simulink model "Eas_Integrated_Harness"  (R2021a)
settings: Solver=FixedStepDiscrete  StartTime=0.0  StopTime=inf  FixedStep=0.01  RelTol=1e-3
settings Model: DataDictionary=DPF_Data_Dictionary.sldd  Creator=SOMNATH  LastModifiedBy=SOMNATH
settings OptimizationCC: BlockReduction=off  DefaultParameterBehavior=Inlined  UseDivisionForNetSlopeComputation=on  EnhancedBackFolding=on  PassReuseOutputArgsAs=Individual arguments  EfficientFloat2IntCast=on  LifeSpan=Inf  OptimizeBlockOrder=speed  DifferentSizesBufferReuse=on  OptimizationCustomize=off  EfficientTunableParamExpr=on
settings DebuggingCC: SignalInfNanChecking=error  SignalRangeChecking=error  ReadBeforeWriteMsg=EnableAllAsError  WriteAfterWriteMsg=EnableAllAsError  WriteAfterReadMsg=EnableAllAsError  AlgebraicLoopMsg=error  ArtificialAlgebraicLoopMsg=error  SaveWithDisabledLinksMsg=error  SaveWithParameterizedLinksMsg=error  BlockPriorityViolationMsg=error  SolverPrmCheckMsg=error  InheritedTsInSrcMsg=error  SingleTaskRateTransMsg=error  TasksWithSamePriorityMsg=error  SigSpecEnsureSampleTimeMsg=error  CheckMatrixSingularityMsg=error  IntegerOverflowMsg=error  ParameterUnderflowMsg=error  ParameterPrecisionLossMsg=error  ParameterTunabilityLossMsg=error  UnderSpecifiedDataTypeMsg=error  UnnecessaryDatatypeConvMsg=warning  VectorMatrixConversionMsg=error  SignalLabelMismatchMsg=error  UnconnectedInputMsg=error  UnconnectedOutputMsg=error  UnconnectedLineMsg=error  SFcnCompatibilityMsg=error  UniqueDataStoreMsg=error  BusObjectLabelMismatch=error  RootOutportRequireBusObject=error  AssertControl=DisableAll  ModelReferenceIOMsg=error  ModelReferenceIOMismatchMessage=error  UnknownTsInhSupMsg=error  ModelReferenceDataLoggingMessage=error  StateNameClashWarn=warning  StrictBusMsg=ErrorOnBusTreatedAsVector  NonBusSignalsTreatedAsBus=error  SFInvalidInputDataAccessInChartInitDiag=error  SFTransitionOutsideNaturalParentDiag=error  SFUnreachableExecutionPathDiag=error  SFUndirectedBroadcastEventsDiag=error  SFTransitionActionBeforeConditionDiag=error  SFTemporalDelaySmallerThanSampleTimeDiag=error  SFSelfTransitionDiag=error  SFExecutionAtInitializationDiag=error  IntegerSaturationMsg=error
settings SFSimCC: CompileTimeRecursionLimit=0  EnableRuntimeRecursion=off  MATLABDynamicMemAlloc=off
settings RTWCC: SystemTargetFile=ert.tlc  GenCodeOnly=on  TemplateMakefile=ert_default_tmf  GenerateReport=on  Toolchain=MinGW64 | gmake (64-bit Windows)  IncludeHyperlinkInReport=on  LaunchReport=on  GenerateTraceInfo=on  GenerateTraceReport=on  GenerateTraceReportSl=on  GenerateTraceReportSf=on  GenerateTraceReportEml=on  GenerateWebview=on  GenerateCodeReplacementReport=on
settings CodeAppCC: ForceParamTrailComments=on  IgnoreCustomStorageClasses=off  OperatorAnnotations=on  SimulinkDataObjDesc=on  SFDataObjDesc=on  MATLABFcnDesc=on  MangleLength=4  InsertBlockDesc=on  ReqsInCode=on
settings ERTTargetCC: TargetLangStandard=C99 (ISO)  UtilityFuncGeneration=Shared location  GenerateSampleERTMain=on  IncludeMdlTerminateFcn=off  SuppressErrorStatus=on  SupportAbsoluteTime=off  SupportNonFinite=off  ParenthesesLevel=Maximum  CastingMode=Standards  GenerateSharedConstants=off  InlinedParameterPlacement=NonHierarchical  ERTCustomFileTemplate=example_file_process.tlc  PreserveExpressionOrder=on  EnableSignedLeftShifts=off  EnableSignedRightShifts=off
settings ConfigComp: CovMetricSettings=dcmwe  DVMode=PropertyProving  DVTestSuiteOptimization=Auto  DVDetectDeadLogic=on  DVDetectActiveLogic=on  DVDetectOutOfBounds=on  DVDetectInfNaN=on  DVDesignMinMaxCheck=on  DVDetectDSMAccessViolations=on  DVDetectHISMViolationsHisl_0002=on  DVDetectHISMViolationsHisl_0003=on  DVDetectHISMViolationsHisl_0004=on  DVDetectHISMViolationsHisl_0028=on  DVDetectBlockInputRangeViolations=on  DVSaveExpectedOutput=on  DVRandomizeNoEffectData=on  DVSaveHarnessModel=on

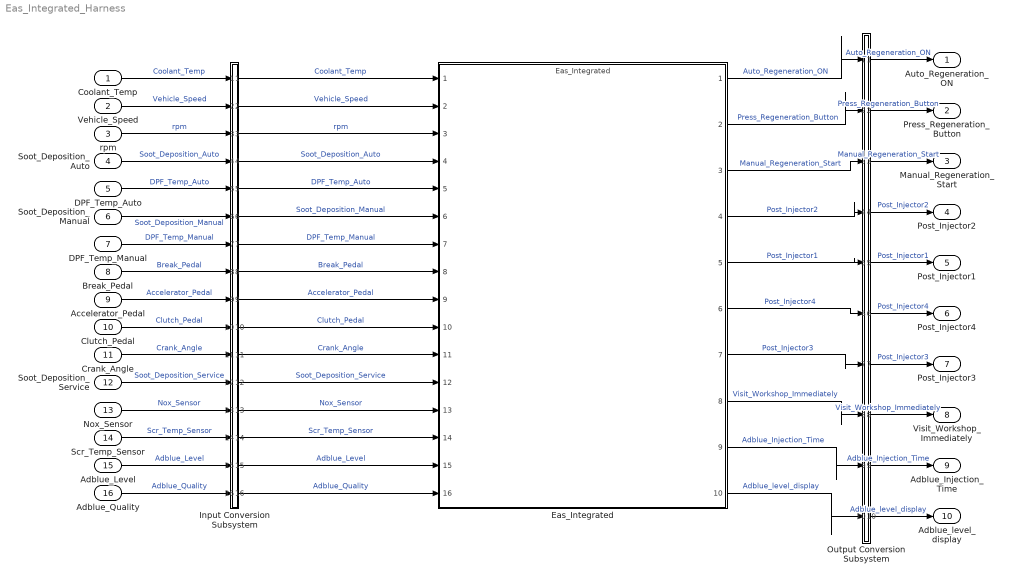
== system Eas_Integrated_Harness ==
  Coolant_Temp : Inport  OutDataTypeStr=int16  PortDimensions=[1]  SampleTime=0.01
  Vehicle_Speed : Inport  Port=2  OutDataTypeStr=uint8  PortDimensions=[1]  SampleTime=0.01
  rpm : Inport  Port=3  OutDataTypeStr=uint16  PortDimensions=[1]  SampleTime=0.01
  Soot_Deposition_Auto : Inport  Port=4  OutDataTypeStr=uint8  PortDimensions=[1]  SampleTime=0.01
  DPF_Temp_Auto : Inport  Port=5  OutDataTypeStr=uint8  PortDimensions=[1]  SampleTime=0.01
  Soot_Deposition_Manual : Inport  Port=6  OutDataTypeStr=uint8  PortDimensions=[1]  SampleTime=0.01
  DPF_Temp_Manual : Inport  Port=7  OutDataTypeStr=int16  PortDimensions=[1]  SampleTime=0.01
  Break_Pedal : Inport  Port=8  OutDataTypeStr=boolean  PortDimensions=[1]  SampleTime=0.01
  Accelerator_Pedal : Inport  Port=9  OutDataTypeStr=boolean  PortDimensions=[1]  SampleTime=0.01
  Clutch_Pedal : Inport  Port=10  OutDataTypeStr=boolean  PortDimensions=[1]  SampleTime=0.01
  Crank_Angle : Inport  Port=11  OutDataTypeStr=uint16  PortDimensions=[1]  SampleTime=0.01
  Soot_Deposition_Service : Inport  Port=12  OutDataTypeStr=uint8  PortDimensions=[1]  SampleTime=0.01
  Nox_Sensor : Inport  Port=13  OutDataTypeStr=uint16  PortDimensions=[1]  SampleTime=0.01
  Scr_Temp_Sensor : Inport  Port=14  OutDataTypeStr=uint16  PortDimensions=[1]  SampleTime=0.01
  Adblue_Level : Inport  Port=15  OutDataTypeStr=uint8  PortDimensions=[1]  SampleTime=0.01
  Adblue_Quality : Inport  Port=16  OutDataTypeStr=double  PortDimensions=[1]  SampleTime=0.01
  Eas_Integrated : ModelReference  ModelNameDialog=Eas_Integrated  SimulationMode=Normal  ModelReferenceVersion=1.57
  Input Conversion Subsystem : Subsystem  Tag=__SLT_ICS__  Description=|
      | Signal spec.
      | and routing
      settings: AttributesFormatString=%<Description>
  Output Conversion Subsystem : Subsystem  Tag=__SLT_OCS__  Description=|
      | Signal spec.
      | and routing
      settings: AttributesFormatString=%<Description>
  Auto_Regeneration_ON : Outport
  Press_Regeneration_Button : Outport  Port=2
  Manual_Regeneration_Start : Outport  Port=3
  Post_Injector2 : Outport  Port=4
  Post_Injector1 : Outport  Port=5
  Post_Injector4 : Outport  Port=6
  Post_Injector3 : Outport  Port=7
  Visit_Workshop_Immediately : Outport  Port=8
  Adblue_Injection_Time : Outport  Port=9
  Adblue_level_display : Outport  Port=10
  wires:
  Coolant_Temp/1 -> Input Conversion Subsystem/1(Inport_1)  "Coolant_Temp"
  Vehicle_Speed/1 -> Input Conversion Subsystem/2(Inport_2)  "Vehicle_Speed"
  rpm/1 -> Input Conversion Subsystem/3(Inport_3)  "rpm"
  Soot_Deposition_Auto/1 -> Input Conversion Subsystem/4(Inport_4)  "Soot_Deposition_Auto"
  DPF_Temp_Auto/1 -> Input Conversion Subsystem/5(Inport_5)  "DPF_Temp_Auto"
  Soot_Deposition_Manual/1 -> Input Conversion Subsystem/6(Inport_6)  "Soot_Deposition_Manual"
  DPF_Temp_Manual/1 -> Input Conversion Subsystem/7(Inport_7)  "DPF_Temp_Manual"
  Break_Pedal/1 -> Input Conversion Subsystem/8(Inport_8)  "Break_Pedal"
  Accelerator_Pedal/1 -> Input Conversion Subsystem/9(Inport_9)  "Accelerator_Pedal"
  Clutch_Pedal/1 -> Input Conversion Subsystem/10(Inport_10)  "Clutch_Pedal"
  Crank_Angle/1 -> Input Conversion Subsystem/11(Inport_11)  "Crank_Angle"
  Soot_Deposition_Service/1 -> Input Conversion Subsystem/12(Inport_12)  "Soot_Deposition_Service"
  Nox_Sensor/1 -> Input Conversion Subsystem/13(Inport_13)  "Nox_Sensor"
  Scr_Temp_Sensor/1 -> Input Conversion Subsystem/14(Inport_14)  "Scr_Temp_Sensor"
  Adblue_Level/1 -> Input Conversion Subsystem/15(Inport_15)  "Adblue_Level"
  Adblue_Quality/1 -> Input Conversion Subsystem/16(Inport_16)  "Adblue_Quality"
  Output Conversion Subsystem/1(Outport_1) -> Auto_Regeneration_ON/1  "Auto_Regeneration_ON"
  Output Conversion Subsystem/2(Outport_2) -> Press_Regeneration_Button/1  "Press_Regeneration_Button"
  Output Conversion Subsystem/3(Outport_3) -> Manual_Regeneration_Start/1  "Manual_Regeneration_Start"
  Output Conversion Subsystem/4(Outport_4) -> Post_Injector2/1  "Post_Injector2"
  Output Conversion Subsystem/5(Outport_5) -> Post_Injector1/1  "Post_Injector1"
  Output Conversion Subsystem/6(Outport_6) -> Post_Injector4/1  "Post_Injector4"
  Output Conversion Subsystem/7(Outport_7) -> Post_Injector3/1  "Post_Injector3"
  Output Conversion Subsystem/8(Outport_8) -> Visit_Workshop_Immediately/1  "Visit_Workshop_Immediately"
  Output Conversion Subsystem/9(Outport_9) -> Adblue_Injection_Time/1  "Adblue_Injection_Time"
  Output Conversion Subsystem/10(Outport_10) -> Adblue_level_display/1  "Adblue_level_display"
  Input Conversion Subsystem/1(Outport_1) -> Eas_Integrated/1  "Coolant_Temp"
  Input Conversion Subsystem/2(Outport_2) -> Eas_Integrated/2  "Vehicle_Speed"
  Input Conversion Subsystem/3(Outport_3) -> Eas_Integrated/3  "rpm"
  Input Conversion Subsystem/4(Outport_4) -> Eas_Integrated/4  "Soot_Deposition_Auto"
  Input Conversion Subsystem/5(Outport_5) -> Eas_Integrated/5  "DPF_Temp_Auto"
  Input Conversion Subsystem/6(Outport_6) -> Eas_Integrated/6  "Soot_Deposition_Manual"
  Input Conversion Subsystem/7(Outport_7) -> Eas_Integrated/7  "DPF_Temp_Manual"
  Input Conversion Subsystem/8(Outport_8) -> Eas_Integrated/8  "Break_Pedal"
  Input Conversion Subsystem/9(Outport_9) -> Eas_Integrated/9  "Accelerator_Pedal"
  Input Conversion Subsystem/10(Outport_10) -> Eas_Integrated/10  "Clutch_Pedal"
  Input Conversion Subsystem/11(Outport_11) -> Eas_Integrated/11  "Crank_Angle"
  Input Conversion Subsystem/12(Outport_12) -> Eas_Integrated/12  "Soot_Deposition_Service"
  Input Conversion Subsystem/13(Outport_13) -> Eas_Integrated/13  "Nox_Sensor"
  Input Conversion Subsystem/14(Outport_14) -> Eas_Integrated/14  "Scr_Temp_Sensor"
  Input Conversion Subsystem/15(Outport_15) -> Eas_Integrated/15  "Adblue_Level"
  Input Conversion Subsystem/16(Outport_16) -> Eas_Integrated/16  "Adblue_Quality"
  Eas_Integrated/1 -> Output Conversion Subsystem/1(Inport_1)  "Auto_Regeneration_ON"
  Eas_Integrated/2 -> Output Conversion Subsystem/2(Inport_2)  "Press_Regeneration_Button"
  Eas_Integrated/3 -> Output Conversion Subsystem/3(Inport_3)  "Manual_Regeneration_Start"
  Eas_Integrated/4 -> Output Conversion Subsystem/4(Inport_4)  "Post_Injector2"
  Eas_Integrated/5 -> Output Conversion Subsystem/5(Inport_5)  "Post_Injector1"
  Eas_Integrated/6 -> Output Conversion Subsystem/6(Inport_6)  "Post_Injector4"
  Eas_Integrated/7 -> Output Conversion Subsystem/7(Inport_7)  "Post_Injector3"
  Eas_Integrated/8 -> Output Conversion Subsystem/8(Inport_8)  "Visit_Workshop_Immediately"
  Eas_Integrated/9 -> Output Conversion Subsystem/9(Inport_9)  "Adblue_Injection_Time"
  Eas_Integrated/10 -> Output Conversion Subsystem/10(Inport_10)  "Adblue_level_display"

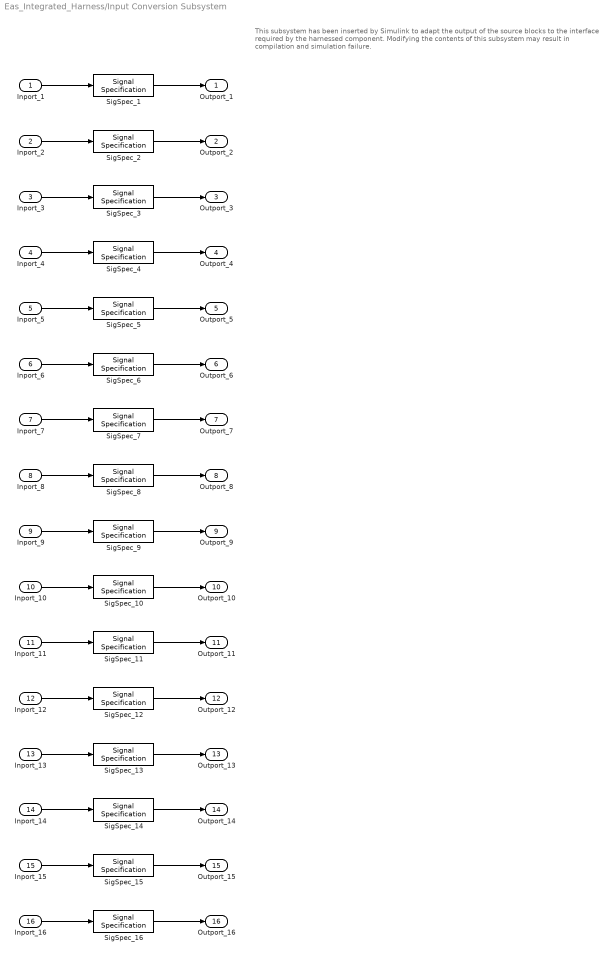
== system Eas_Integrated_Harness/Input Conversion Subsystem ==
  note: This subsystem has been inserted by Simulink to adapt the output of the source blocks to the interface required by the harnessed component.
      |  Modifying the contents of this subsystem may result in compilation and simulation failure.
  Inport_1 : Inport
  Inport_2 : Inport  Port=2
  Inport_3 : Inport  Port=3
  Inport_4 : Inport  Port=4
  Inport_5 : Inport  Port=5
  Inport_6 : Inport  Port=6
  Inport_7 : Inport  Port=7
  Inport_8 : Inport  Port=8
  Inport_9 : Inport  Port=9
  Inport_10 : Inport  Port=10
  Inport_11 : Inport  Port=11
  Inport_12 : Inport  Port=12
  Inport_13 : Inport  Port=13
  Inport_14 : Inport  Port=14
  Inport_15 : Inport  Port=15
  Inport_16 : Inport  Port=16
  SigSpec_1 : SignalSpecification  OutDataTypeStr=int16  Dimensions=[1]  SampleTime=0.01
  SigSpec_10 : SignalSpecification  OutDataTypeStr=boolean  Dimensions=[1]  SampleTime=0.01
  SigSpec_{3,11,13..14} (4 alike) : SignalSpecification  OutDataTypeStr=uint16  Dimensions=[1]  SampleTime=0.01
  SigSpec_{2,4..6,12,15} (6 alike) : SignalSpecification  OutDataTypeStr=uint8  Dimensions=[1]  SampleTime=0.01
  SigSpec_16 : SignalSpecification  OutDataTypeStr=double  Dimensions=[1]  SampleTime=0.01
  SigSpec_7 : SignalSpecification  OutDataTypeStr=int16  Dimensions=[1]  SampleTime=0.01
  SigSpec_8 : SignalSpecification  OutDataTypeStr=boolean  Dimensions=[1]  SampleTime=0.01
  SigSpec_9 : SignalSpecification  OutDataTypeStr=boolean  Dimensions=[1]  SampleTime=0.01
  Outport_1 : Outport
  Outport_2 : Outport  Port=2
  Outport_3 : Outport  Port=3
  Outport_4 : Outport  Port=4
  Outport_5 : Outport  Port=5
  Outport_6 : Outport  Port=6
  Outport_7 : Outport  Port=7
  Outport_8 : Outport  Port=8
  Outport_9 : Outport  Port=9
  Outport_10 : Outport  Port=10
  Outport_11 : Outport  Port=11
  Outport_12 : Outport  Port=12
  Outport_13 : Outport  Port=13
  Outport_14 : Outport  Port=14
  Outport_15 : Outport  Port=15
  Outport_16 : Outport  Port=16
  wires:
  SigSpec_1/1 -> Outport_1/1
  Inport_1/1 -> SigSpec_1/1
  SigSpec_2/1 -> Outport_2/1
  Inport_2/1 -> SigSpec_2/1
  SigSpec_3/1 -> Outport_3/1
  Inport_3/1 -> SigSpec_3/1
  SigSpec_4/1 -> Outport_4/1
  Inport_4/1 -> SigSpec_4/1
  SigSpec_5/1 -> Outport_5/1
  Inport_5/1 -> SigSpec_5/1
  SigSpec_6/1 -> Outport_6/1
  Inport_6/1 -> SigSpec_6/1
  SigSpec_7/1 -> Outport_7/1
  Inport_7/1 -> SigSpec_7/1
  SigSpec_8/1 -> Outport_8/1
  Inport_8/1 -> SigSpec_8/1
  SigSpec_9/1 -> Outport_9/1
  Inport_9/1 -> SigSpec_9/1
  SigSpec_10/1 -> Outport_10/1
  Inport_10/1 -> SigSpec_10/1
  SigSpec_11/1 -> Outport_11/1
  Inport_11/1 -> SigSpec_11/1
  SigSpec_12/1 -> Outport_12/1
  Inport_12/1 -> SigSpec_12/1
  SigSpec_13/1 -> Outport_13/1
  Inport_13/1 -> SigSpec_13/1
  SigSpec_14/1 -> Outport_14/1
  Inport_14/1 -> SigSpec_14/1
  SigSpec_15/1 -> Outport_15/1
  Inport_15/1 -> SigSpec_15/1
  SigSpec_16/1 -> Outport_16/1
  Inport_16/1 -> SigSpec_16/1

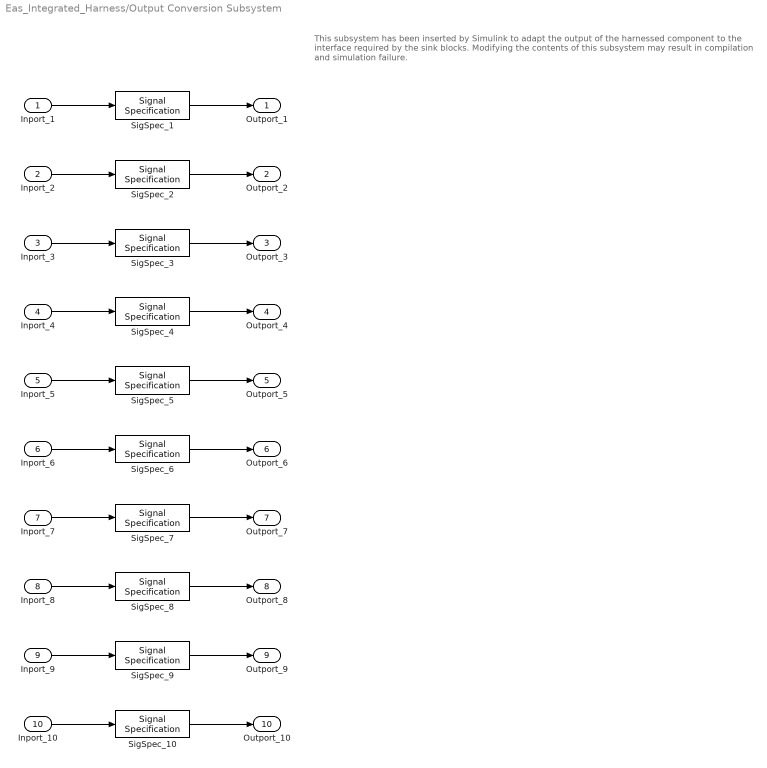
== system Eas_Integrated_Harness/Output Conversion Subsystem ==
  note: This subsystem has been inserted by Simulink to adapt the output of the harnessed component to the interface required by the sink blocks.
      |  Modifying the contents of this subsystem may result in compilation and simulation failure.
  Inport_1 : Inport
  Inport_2 : Inport  Port=2
  Inport_3 : Inport  Port=3
  Inport_4 : Inport  Port=4
  Inport_5 : Inport  Port=5
  Inport_6 : Inport  Port=6
  Inport_7 : Inport  Port=7
  Inport_8 : Inport  Port=8
  Inport_9 : Inport  Port=9
  Inport_10 : Inport  Port=10
  SigSpec_{1..8} (8 alike) : SignalSpecification  OutDataTypeStr=boolean  Dimensions=[1]  SampleTime=0.01
  SigSpec_10 : SignalSpecification  OutDataTypeStr=Enum: adblue_capacity  Dimensions=[1]  SampleTime=0.01
  SigSpec_9 : SignalSpecification  OutDataTypeStr=double  Dimensions=[1]  SampleTime=0.01
  Outport_1 : Outport
  Outport_2 : Outport  Port=2
  Outport_3 : Outport  Port=3
  Outport_4 : Outport  Port=4
  Outport_5 : Outport  Port=5
  Outport_6 : Outport  Port=6
  Outport_7 : Outport  Port=7
  Outport_8 : Outport  Port=8
  Outport_9 : Outport  Port=9
  Outport_10 : Outport  Port=10
  wires:
  Inport_1/1 -> SigSpec_1/1
  SigSpec_1/1 -> Outport_1/1
  Inport_2/1 -> SigSpec_2/1
  SigSpec_2/1 -> Outport_2/1
  Inport_3/1 -> SigSpec_3/1
  SigSpec_3/1 -> Outport_3/1
  Inport_4/1 -> SigSpec_4/1
  SigSpec_4/1 -> Outport_4/1
  Inport_5/1 -> SigSpec_5/1
  SigSpec_5/1 -> Outport_5/1
  Inport_6/1 -> SigSpec_6/1
  SigSpec_6/1 -> Outport_6/1
  Inport_7/1 -> SigSpec_7/1
  SigSpec_7/1 -> Outport_7/1
  Inport_8/1 -> SigSpec_8/1
  SigSpec_8/1 -> Outport_8/1
  Inport_9/1 -> SigSpec_9/1
  SigSpec_9/1 -> Outport_9/1
  Inport_10/1 -> SigSpec_10/1
  SigSpec_10/1 -> Outport_10/1
